simulink model "gridv1"  (R2021a)
settings: Solver=VariableStepAuto  StartTime=0.0  StopTime=inf  RelTol=1e-3
libraries: spsThreePhaseBreakerLib x12, spsMosfetLib x12, spsThreePhaseSeriesRLCLoadLib x10, spsMeanLib x6, pid_lib x5, simulink x4, spsPLL3phLib x4, spsThreePhaseVIMeasurementLib x4, spsAsynchronousMachineSIUnitsLib x2, spsDCVoltageSourceLib x2, spsFourierLib x2, spsGroundLib x2
(part 1 of 2)
settings Model: SimulationMode=accelerator  Creator=Ramadan B.M.S  LastModifiedBy=Ramadan B.M.S
settings SolverCC: ZeroCrossAlgorithm=Adaptive  AutoInsertRateTranBlk=on
settings DebuggingCC: IgnoredZcDiagnostic=none

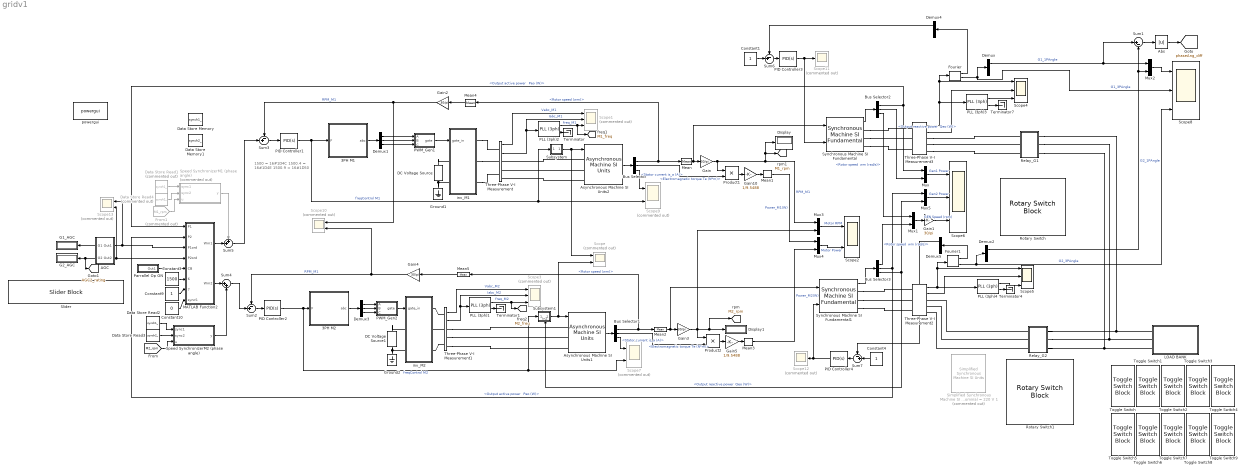
== system gridv1 ==
  note: 1500 = 16#1D4C
      | 1500.4 = 16#1D4E
      | 1500.9 = 16#1D50
  3PH M1 : Subsystem
  3PH M2 : Subsystem
  AGC : Subsystem
      settings: PortSchema="{\"entries\":[{\"content\":{\"sides\":[{\"content\":{\"connectorIds\":[\"Out3\",\"Out4\"]},\"type\":\"ConnectorPlacement.EquallySpacedRectSide\",\"uuid\":\"0458f88f-2a90-4e9d-a6e7-72d7481f8c74\"},{\"content\":{\"connectorIds\":[\"Out1\",\"Out2\"],\"side\":\"RIGHT\"},\"type\":\"ConnectorPlacement.EquallySpacedRectSide\",\"uuid\":\"40e75e7a-a838-46b0-adb7-8af141426c13\"},{\"content\":{\"connectorIds\":[],\"side\":\"TOP\"},\"type\":\"ConnectorPlacement.EquallySpacedRectSide\",\"uuid\":\"7ac7dab2-5483-477d-b4b4-330f83a557ce\"}]},\"type\":\"ConnectorPlacement.EquallySpacedConnector\",\"uuid\":\"5bf97401-9b0d-4cd2-ac22-a4057234a7d6\"}],\"packageUris\":[\"http://schema.mathworks.com/mf0/Connector/R2020b\"],\"version\":\"1.0\"}"
  Abs : Abs
  Asynchronous Machine SI Units1 : spsAsynchronousMachineSIUnitsLib/Asynchronous Machine SI Units  RotorType=Squirrel-cage  PresetModel="17:  20 HP (15KW)   400 V 50Hz 1460 RPM"  MechanicalLoad=Torque Tm  ShowDetailedParameters=on  ReferenceFrame=Rotor  Units=SI  MeasurementBus=off  NominalParameters=[1.5e+04 400 50]  VoltageRatio=1  Stator=[0.2147 0.000991]  Rotor=[0.2205 0.000991]  Cage1=[0.4155 0.002066]  Cage2=[0.4168 0.0003495]  Lm=0.06419  Mechanical=[0.102 0.009541 2]  PolePairs=2  InitialConditions=[0 0 0 0 0 0 0 0]  SimulateSaturation=off  Saturation=[14.03593122, 27.81365428, 53.79336849, 72.68890987, 97.98006896, 148.6815601, 215.7428561, 302.9841135, 428.7778367 ; 230, 322, 414, 460, 506, 552, 598, 644, 690]  LoadFlowParameters=1492000  TsPowergui=0  TsBlock=-1  IterativeModel=Trapezoidal non iterative  IterativeDiscreteModel=Trapezoidal robust  Pmec=0  mask(Asynchronous Machine){}
      mask Display: image('M2.jpg'); % Use "Edit Image" on toolstrip to change.
  Asynchronous Machine SI Units2 : spsAsynchronousMachineSIUnitsLib/Asynchronous Machine SI Units  RotorType=Squirrel-cage  PresetModel="17:  20 HP (15KW)   400 V 50Hz 1460 RPM"  MechanicalLoad=Torque Tm  ShowDetailedParameters=on  ReferenceFrame=Rotor  Units=SI  MeasurementBus=off  NominalParameters=[1.5e+04 400 50]  VoltageRatio=1  Stator=[0.2147 0.000991]  Rotor=[0.2205 0.000991]  Cage1=[0.4155 0.002066]  Cage2=[0.4168 0.0003495]  Lm=0.06419  Mechanical=[0.102 0.009541 2]  PolePairs=2  InitialConditions=[0 0 0 0 0 0 0 0]  SimulateSaturation=off  Saturation=[14.03593122, 27.81365428, 53.79336849, 72.68890987, 97.98006896, 148.6815601, 215.7428561, 302.9841135, 428.7778367 ; 230, 322, 414, 460, 506, 552, 598, 644, 690]  LoadFlowParameters=1492000  TsPowergui=0  TsBlock=-1  IterativeModel=Trapezoidal non iterative  IterativeDiscreteModel=Trapezoidal robust  Pmec=0  mask(Asynchronous Machine){}
      mask Display: image('M1.jpg'); % Use "Edit Image" on toolstrip to change.
  Bus Selector : BusSelector  OutputSignals=Mechanical.Rotor speed (wm),Mechanical.Electromagnetic torque Te (N*m),Stator measurements.Stator current is_a (A)
  Bus Selector1 : BusSelector  OutputSignals=Mechanical.Rotor speed (wm),Mechanical.Electromagnetic torque Te (N*m),Stator measurements.Stator current is_a (A)
  Bus Selector2 : BusSelector  OutputSignals="Output active power   Peo (W),Output reactive power  Qeo (W),Mechanical.Rotor speed  wm (rad/s)"
  Bus Selector3 : BusSelector  OutputSignals="Mechanical.Rotor speed  wm (rad/s),Output active power   Peo (W),Output reactive power  Qeo (W)"
  Constant1 : Constant
  Constant10 : Constant  Value=0
  Constant3 : Constant  Value=1500
  Constant4 : Constant
  Constant9 : Constant
  DC Voltage Source : spsDCVoltageSourceLib/DC Voltage Source  Amplitude=566  Measurements=None
  DC Voltage Source1 : spsDCVoltageSourceLib/DC Voltage Source  Amplitude=566  Measurements=None
  Data Store Memory : DataStoreMemory  DataStoreName=synch1_  ReadBeforeWriteMsg=warning  WriteAfterWriteMsg=warning  WriteAfterReadMsg=warning  ShowAdditionalParam=off
  Data Store Memory1 : DataStoreMemory  DataStoreName=synch2_  ReadBeforeWriteMsg=warning  WriteAfterWriteMsg=warning  WriteAfterReadMsg=warning  ShowAdditionalParam=off
  Data Store Read1 : DataStoreRead  Commented=on  DataStoreName=synch1_  IndexOptions=Index vector (dialog)  Indices=1  OutputSizes=1
  Data Store Read2 : DataStoreRead  DataStoreName=synch1_  IndexOptions=Index vector (dialog)  Indices=1  OutputSizes=1
  Data Store Read3 : DataStoreRead  DataStoreName=synch2_  IndexOptions=Index vector (dialog)  Indices=1  OutputSizes=1
  Data Store Read4 : DataStoreRead  Commented=on  DataStoreName=synch2_  IndexOptions=Index vector (dialog)  Indices=1  OutputSizes=1
  Demux{,1..5} (6 alike) : Demux  Outputs=3
  Display : Display
  Display1 : Display
  Fourier : spsFourierLib/Fourier  Freq=50  n=1  InInit=[0, 0]  Ts=0
      settings: SourceProductBaseCode=PS
  Fourier1 : spsFourierLib/Fourier  Freq=50  n=1  InInit=[0, 0]  Ts=0
      settings: SourceProductBaseCode=PS
  From1 : From  Commented=on  GotoTag=M1_rpm  TagVisibility=global
  G1_AGC : Display
      settings: Decimation=100
  G2_AGC : Display
      settings: Decimation=100
  Gain{,1..4} (5 alike) : Gain  Gain=30/pi
  Gain10 : Gain  Gain=1/9.5488
  Gain5 : Gain  Gain=1/9.5488
  Ground1 : spsGroundLib/Ground  LConnTagsString=a
  Ground2 : spsGroundLib/Ground  LConnTagsString=a
  LOAD BANK : Subsystem
  MATLAB Function2 : MATLAB Function  TreatAsAtomicUnit=on
  Mean{,1..3} (4 alike) : spsMeanLib/Mean  Freq=1  Vinit=0  Ts=0
  Mean4 : spsMeanLib/Mean  Freq=10  Vinit=0  Ts=0
  Mean5 : spsMeanLib/Mean  Freq=10  Vinit=0  Ts=0
  Mux{,1..5} (6 alike) : Mux  Inputs=2
  PID Controller1 : pid_lib/PID Controller  Controller=PID  Form=Parallel  TimeDomain=Continuous-time  UseExternalTs=off  SampleTime=-1  IntegratorMethod=Forward Euler  FilterMethod=Forward Euler  ControllerParametersSource=internal  P=0.06  I=0.12  D=0  UseFilter=on  N=100  TunerSelectOption=Transfer Function Based (PID Tuner App)  ZeroCross=off  InitialConditionSource=internal  InitialConditionForIntegrator=0  InitialConditionForFilter=0  DifferentiatorICPrevScaledInput=0  ExternalReset=none  TrackingMode=off  Kt=1  LimitOutput=on  SatLimitsSource=internal  UpperSaturationLimit=52.5  LowerSaturationLimit=0  LinearizeAsGain=on  AntiWindupMode=back-calculation  Kb=1  POutMin=[]  POutMax=[]  IOutMin=[]  IOutMax=[]  DOutMin=[]  DOutMax=[]  NOutMin=[]  NOutMax=[]  SumOutMin=[]  SumOutMax=[]  SaturationOutMin=[]  SaturationOutMax=[]  PParamMin=[]  PParamMax=[]  IParamMin=[]  IParamMax=[]  DParamMin=[]  DParamMax=[]  NParamMin=[]  NParamMax=[]  KbParamMin=[]  KbParamMax=[]  KtParamMin=[]  KtParamMax=[]  KbOutMin=[]  KbOutMax=[]  KtOutMin=[]  KtOutMax=[]  IntegratorOutMin=[]  IntegratorOutMax=[]  FilterOutMin=[]  FilterOutMax=[]  SumI1OutMin=[]  SumI1OutMax=[]  SumI2OutMin=[]  SumI2OutMax=[]  SumI3OutMin=[]  SumI3OutMax=[]  SumI4OutMin=[]  SumI4OutMax=[]  SumDOutMin=[]  SumDOutMax=[]  DifferentiatorOutMin=[]  DifferentiatorOutMax=[]  FilterDiffOutCoefMin=[]  FilterDiffOutCoefMax=[]  ReciprocalOutMin=[]  ReciprocalOutMax=[]  SumDenOutMin=[]  SumDenOutMax=[]  SumNumOutMin=[]  SumNumOutMax=[]  DivideOutMin=[]  DivideOutMax=[]  UdiffTsProdOutMin=[]  UdiffTsProdOutMax=[]  NTsProdOutMin=[]  NTsProdOutMax=[]  UintegralTsProdOutMin=[]  UintegralTsProdOutMax=[]  UngainTsProdOutMin=[]  UngainTsProdOutMax=[]  IntegratorContinuousStateAttributes=''  IntegratorStateMustResolveToSignalObject=off  IntegratorRTWStateStorageClass=Auto  FilterContinuousStateAttributes=''  FilterStateMustResolveToSignalObject=off  FilterRTWStateStorageClass=Auto  ParallelPVariant=InternalParameters  IdealPVariant=Disabled  IVariant=InternalParameters  DVariant=InternalParameters  IntegratorVariant=Continuous  SatVariant=Enabled  AWVariant=BackCalculation  PCopyVariant=Disabled  TRVariant=Disabled  FdbkBlocksVariant=Forward  IdealPFdbkVariant=Disabled  SatFdbkVariant=Disabled  DerivativeFilterVariant=ContFilter  NVariant=InternalParameters  NCopyVariant=Disabled  FilterICVariant=InternalICsFilter  IntegratorICVariant=InternalICs  ExternalResetVariant=Disabled  TRSumVariant=Passthrough  SumFdbkVariant=Disabled  SumVariant=Sum_PID  TsampFilterVariant=InternalTs  TsampNgainVariant=Passthrough  TsampIntegralVariant=Passthrough  ExternalSaturationOutDataTypeStr=Inherit: Same as second input
  PID Controller2 : pid_lib/PID Controller  Controller=PID  Form=Parallel  TimeDomain=Continuous-time  UseExternalTs=off  SampleTime=-1  IntegratorMethod=Forward Euler  FilterMethod=Forward Euler  ControllerParametersSource=internal  P=0.06  I=0.12  D=0  UseFilter=on  N=100  TunerSelectOption=Transfer Function Based (PID Tuner App)  ZeroCross=off  InitialConditionSource=internal  InitialConditionForIntegrator=0  InitialConditionForFilter=0  DifferentiatorICPrevScaledInput=0  ExternalReset=none  TrackingMode=off  Kt=1  LimitOutput=on  SatLimitsSource=internal  UpperSaturationLimit=52.5  LowerSaturationLimit=0  LinearizeAsGain=on  AntiWindupMode=back-calculation  Kb=1  POutMin=[]  POutMax=[]  IOutMin=[]  IOutMax=[]  DOutMin=[]  DOutMax=[]  NOutMin=[]  NOutMax=[]  SumOutMin=[]  SumOutMax=[]  SaturationOutMin=[]  SaturationOutMax=[]  PParamMin=[]  PParamMax=[]  IParamMin=[]  IParamMax=[]  DParamMin=[]  DParamMax=[]  NParamMin=[]  NParamMax=[]  KbParamMin=[]  KbParamMax=[]  KtParamMin=[]  KtParamMax=[]  KbOutMin=[]  KbOutMax=[]  KtOutMin=[]  KtOutMax=[]  IntegratorOutMin=[]  IntegratorOutMax=[]  FilterOutMin=[]  FilterOutMax=[]  SumI1OutMin=[]  SumI1OutMax=[]  SumI2OutMin=[]  SumI2OutMax=[]  SumI3OutMin=[]  SumI3OutMax=[]  SumI4OutMin=[]  SumI4OutMax=[]  SumDOutMin=[]  SumDOutMax=[]  DifferentiatorOutMin=[]  DifferentiatorOutMax=[]  FilterDiffOutCoefMin=[]  FilterDiffOutCoefMax=[]  ReciprocalOutMin=[]  ReciprocalOutMax=[]  SumDenOutMin=[]  SumDenOutMax=[]  SumNumOutMin=[]  SumNumOutMax=[]  DivideOutMin=[]  DivideOutMax=[]  UdiffTsProdOutMin=[]  UdiffTsProdOutMax=[]  NTsProdOutMin=[]  NTsProdOutMax=[]  UintegralTsProdOutMin=[]  UintegralTsProdOutMax=[]  UngainTsProdOutMin=[]  UngainTsProdOutMax=[]  IntegratorContinuousStateAttributes=''  IntegratorStateMustResolveToSignalObject=off  IntegratorRTWStateStorageClass=Auto  FilterContinuousStateAttributes=''  FilterStateMustResolveToSignalObject=off  FilterRTWStateStorageClass=Auto  ParallelPVariant=InternalParameters  IdealPVariant=Disabled  IVariant=InternalParameters  DVariant=InternalParameters  IntegratorVariant=Continuous  SatVariant=Enabled  AWVariant=BackCalculation  PCopyVariant=Disabled  TRVariant=Disabled  FdbkBlocksVariant=Forward  IdealPFdbkVariant=Disabled  SatFdbkVariant=Disabled  DerivativeFilterVariant=ContFilter  NVariant=InternalParameters  NCopyVariant=Disabled  FilterICVariant=InternalICsFilter  IntegratorICVariant=InternalICs  ExternalResetVariant=Disabled  TRSumVariant=Passthrough  SumFdbkVariant=Disabled  SumVariant=Sum_PID  TsampFilterVariant=InternalTs  TsampNgainVariant=Passthrough  TsampIntegralVariant=Passthrough  ExternalSaturationOutDataTypeStr=Inherit: Same as second input
  PID Controller3 : pid_lib/PID Controller  Controller=PID  Form=Parallel  TimeDomain=Continuous-time  UseExternalTs=off  SampleTime=-1  IntegratorMethod=Forward Euler  FilterMethod=Forward Euler  ControllerParametersSource=internal  P=10  I=17  D=0  UseFilter=on  N=100  TunerSelectOption=Transfer Function Based (PID Tuner App)  ZeroCross=off  InitialConditionSource=internal  InitialConditionForIntegrator=0  InitialConditionForFilter=0  DifferentiatorICPrevScaledInput=0  ExternalReset=none  TrackingMode=off  Kt=1  LimitOutput=on  SatLimitsSource=internal  UpperSaturationLimit=15  LowerSaturationLimit=0  LinearizeAsGain=on  AntiWindupMode=back-calculation  Kb=1  POutMin=[]  POutMax=[]  IOutMin=[]  IOutMax=[]  DOutMin=[]  DOutMax=[]  NOutMin=[]  NOutMax=[]  SumOutMin=[]  SumOutMax=[]  SaturationOutMin=[]  SaturationOutMax=[]  PParamMin=[]  PParamMax=[]  IParamMin=[]  IParamMax=[]  DParamMin=[]  DParamMax=[]  NParamMin=[]  NParamMax=[]  KbParamMin=[]  KbParamMax=[]  KtParamMin=[]  KtParamMax=[]  KbOutMin=[]  KbOutMax=[]  KtOutMin=[]  KtOutMax=[]  IntegratorOutMin=[]  IntegratorOutMax=[]  FilterOutMin=[]  FilterOutMax=[]  SumI1OutMin=[]  SumI1OutMax=[]  SumI2OutMin=[]  SumI2OutMax=[]  SumI3OutMin=[]  SumI3OutMax=[]  SumI4OutMin=[]  SumI4OutMax=[]  SumDOutMin=[]  SumDOutMax=[]  DifferentiatorOutMin=[]  DifferentiatorOutMax=[]  FilterDiffOutCoefMin=[]  FilterDiffOutCoefMax=[]  ReciprocalOutMin=[]  ReciprocalOutMax=[]  SumDenOutMin=[]  SumDenOutMax=[]  SumNumOutMin=[]  SumNumOutMax=[]  DivideOutMin=[]  DivideOutMax=[]  UdiffTsProdOutMin=[]  UdiffTsProdOutMax=[]  NTsProdOutMin=[]  NTsProdOutMax=[]  UintegralTsProdOutMin=[]  UintegralTsProdOutMax=[]  UngainTsProdOutMin=[]  UngainTsProdOutMax=[]  IntegratorContinuousStateAttributes=''  IntegratorStateMustResolveToSignalObject=off  IntegratorRTWStateStorageClass=Auto  FilterContinuousStateAttributes=''  FilterStateMustResolveToSignalObject=off  FilterRTWStateStorageClass=Auto  ParallelPVariant=InternalParameters  IdealPVariant=Disabled  IVariant=InternalParameters  DVariant=InternalParameters  IntegratorVariant=Continuous  SatVariant=Enabled  AWVariant=BackCalculation  PCopyVariant=Disabled  TRVariant=Disabled  FdbkBlocksVariant=Forward  IdealPFdbkVariant=Disabled  SatFdbkVariant=Disabled  DerivativeFilterVariant=ContFilter  NVariant=InternalParameters  NCopyVariant=Disabled  FilterICVariant=InternalICsFilter  IntegratorICVariant=InternalICs  ExternalResetVariant=Disabled  TRSumVariant=Passthrough  SumFdbkVariant=Disabled  SumVariant=Sum_PID  TsampFilterVariant=InternalTs  TsampNgainVariant=Passthrough  TsampIntegralVariant=Passthrough  ExternalSaturationOutDataTypeStr=Inherit: Same as second input
  PID Controller4 : pid_lib/PID Controller  Controller=PID  Form=Parallel  TimeDomain=Continuous-time  UseExternalTs=off  SampleTime=-1  IntegratorMethod=Forward Euler  FilterMethod=Forward Euler  ControllerParametersSource=internal  P=10  I=17  D=0  UseFilter=on  N=100  TunerSelectOption=Transfer Function Based (PID Tuner App)  ZeroCross=off  InitialConditionSource=internal  InitialConditionForIntegrator=0  InitialConditionForFilter=0  DifferentiatorICPrevScaledInput=0  ExternalReset=none  TrackingMode=off  Kt=1  LimitOutput=on  SatLimitsSource=internal  UpperSaturationLimit=15  LowerSaturationLimit=0  LinearizeAsGain=on  AntiWindupMode=back-calculation  Kb=1  POutMin=[]  POutMax=[]  IOutMin=[]  IOutMax=[]  DOutMin=[]  DOutMax=[]  NOutMin=[]  NOutMax=[]  SumOutMin=[]  SumOutMax=[]  SaturationOutMin=[]  SaturationOutMax=[]  PParamMin=[]  PParamMax=[]  IParamMin=[]  IParamMax=[]  DParamMin=[]  DParamMax=[]  NParamMin=[]  NParamMax=[]  KbParamMin=[]  KbParamMax=[]  KtParamMin=[]  KtParamMax=[]  KbOutMin=[]  KbOutMax=[]  KtOutMin=[]  KtOutMax=[]  IntegratorOutMin=[]  IntegratorOutMax=[]  FilterOutMin=[]  FilterOutMax=[]  SumI1OutMin=[]  SumI1OutMax=[]  SumI2OutMin=[]  SumI2OutMax=[]  SumI3OutMin=[]  SumI3OutMax=[]  SumI4OutMin=[]  SumI4OutMax=[]  SumDOutMin=[]  SumDOutMax=[]  DifferentiatorOutMin=[]  DifferentiatorOutMax=[]  FilterDiffOutCoefMin=[]  FilterDiffOutCoefMax=[]  ReciprocalOutMin=[]  ReciprocalOutMax=[]  SumDenOutMin=[]  SumDenOutMax=[]  SumNumOutMin=[]  SumNumOutMax=[]  DivideOutMin=[]  DivideOutMax=[]  UdiffTsProdOutMin=[]  UdiffTsProdOutMax=[]  NTsProdOutMin=[]  NTsProdOutMax=[]  UintegralTsProdOutMin=[]  UintegralTsProdOutMax=[]  UngainTsProdOutMin=[]  UngainTsProdOutMax=[]  IntegratorContinuousStateAttributes=''  IntegratorStateMustResolveToSignalObject=off  IntegratorRTWStateStorageClass=Auto  FilterContinuousStateAttributes=''  FilterStateMustResolveToSignalObject=off  FilterRTWStateStorageClass=Auto  ParallelPVariant=InternalParameters  IdealPVariant=Disabled  IVariant=InternalParameters  DVariant=InternalParameters  IntegratorVariant=Continuous  SatVariant=Enabled  AWVariant=BackCalculation  PCopyVariant=Disabled  TRVariant=Disabled  FdbkBlocksVariant=Forward  IdealPFdbkVariant=Disabled  SatFdbkVariant=Disabled  DerivativeFilterVariant=ContFilter  NVariant=InternalParameters  NCopyVariant=Disabled  FilterICVariant=InternalICsFilter  IntegratorICVariant=InternalICs  ExternalResetVariant=Disabled  TRSumVariant=Passthrough  SumFdbkVariant=Disabled  SumVariant=Sum_PID  TsampFilterVariant=InternalTs  TsampNgainVariant=Passthrough  TsampIntegralVariant=Passthrough  ExternalSaturationOutDataTypeStr=Inherit: Same as second input
  PLL (3ph){1..4} (4 alike) : spsPLL3phLib/PLL (3ph)  Fmin=45  Par_Init=[0, 1]  ParK=[180, 3800, 1]  TcD=1e-4  MaxRateChangeFreq=12  FilterCutOffFreq=25  Ts=0  AGC=on
  PWM_Gen1 : Subsystem
  PWM_Gen2 : Subsystem
  Parrallel Op ON : Subsystem
  Product1 : Product
  Product2 : Product
  Relay_G1 : Subsystem
  Relay_G2 : Subsystem
  Rotary Switch : RotarySwitchBlock
      settings: Values={{'OPEN', 'CLOSE'}, [0 1]}
  Rotary Switch1 : RotarySwitchBlock
      settings: Values={{'OPEN', 'CLOSE'}, [0 1]}
  Scope{,7,9..10,13} (5 alike) : Scope  Commented=on  NumInputPorts=2
  Scope1 : Scope  Commented=on  NumInputPorts=3
  Scope11 : Scope  Commented=on
  Scope12 : Scope  Commented=on
  Scope2 : Scope  NumInputPorts=2
  Scope3 : Scope  Commented=on  NumInputPorts=3
  Scope{4..6,8} (4 alike) : Scope  NumInputPorts=3
  Simplified Synchronous Machine SI Units If nominal  = 1.8 A Xs = 18.85 Ohm a 1800 rpm Ls = 0.05 H Laf = 0.4584 H Ea_LL nominal = 220 V 1 : spsSimplifiedSynchronousMachineSIUnitsLib/Simplified Synchronous Machine SI Units  Commented=on  ConnectionType=3-wire Y  MechanicalLoad=Speed w  MeasurementBus=off  NominalParameters=[15000 400 50]  Mechanical=[1e6 0 2]  InternalRL=[0.01 0.01]  InitialConditions="[ 0,0   0,0,0   0,0,0 ]"  IterativeDiscreteModel=Trapezoidal robust  TsBlock=-1  TsPowergui=0  LoadFlowParameters=[1,0,0,0,0]  Units=1  BusType=PV  Pref=0  Qref=0  Qmin=-inf  Qmax=+inf  PLF=0  QLF=0  mask(Simplified Synchronous Machine){}
      settings: SourceProductBaseCode=PS
      mask Display: image('G2.jpg'); % Use "Edit Image" on toolstrip to change.
  Slider : SliderBlock  TickInterval=10
  Speed SynchronizerM1 (phase angle) : MATLAB Function  Commented=on  TreatAsAtomicUnit=on
  Speed SynchronizerM2 (phase angle) : MATLAB Function  TreatAsAtomicUnit=on
  Subsystem : Subsystem
  Subsystem1 : Subsystem
      settings: PortSchema="{\"entries\":[{\"content\":{\"sides\":[{\"content\":{\"connectorIds\":[\"In1\"]},\"type\":\"ConnectorPlacement.EquallySpacedRectSide\",\"uuid\":\"6fb75f93-f453-4c8c-8eb2-b078f2ee4494\"},{\"content\":{\"connectorIds\":[\"Out1\"],\"side\":\"RIGHT\"},\"type\":\"ConnectorPlacement.EquallySpacedRectSide\",\"uuid\":\"6ec336d8-76a4-4c07-bc41-67ee684e5bd8\"},{\"content\":{\"connectorIds\":[],\"side\":\"TOP\"},\"type\":\"ConnectorPlacement.EquallySpacedRectSide\",\"uuid\":\"24ce01c0-9e7f-4b6f-9b18-6c8c2670b010\"},{\"content\":{\"connectorIds\":[\"In2\"],\"side\":\"BOTTOM\"},\"type\":\"ConnectorPlacement.EquallySpacedRectSide\",\"uuid\":\"901aa75b-c78e-4bda-b9b4-99ea4194a71a\"}]},\"type\":\"ConnectorPlacement.EquallySpacedConnector\",\"uuid\":\"a6afde9e-346d-4066-a3a3-61c85561d5e0\"}],\"packageUris\":[\"http://schema.mathworks.com/mf0/Connector/R2020b\"],\"version\":\"1.0\"}"
  Sum1 : Sum  Inputs=|+-
  Sum{2..3,6..7} (4 alike) : Sum  Inputs=-+|
  Sum4 : Sum  Inputs=|++
  Sum5 : Sum  Inputs=++|
  Synchronous Machine SI Fundamental : spsSynchronousMachineSIFundamentalLib/Synchronous Machine SI Fundamental  PresetModel=02: 50Hz 400V 16kVA 1500RPM  MechanicalLoad=Speed w  ShowDetailedParameters=on  RotorType=Salient-pole  Units=SI fundamental parameters  MeasurementBus=off  NominalParameters=[1.6e+04 400 50]  Stator=[0.645 0.002228 0.05297 0.02518]  Field=[0.3968 0.005492]  Dampers2=[ 0.0664, 1.387e-3, 0.0292, 6.896e-4, 7.907e-3, 2.477e-3]  Dampers1=[0.9843 0.003371 1.545 0.004906]  Mechanical=[0.1278 0.013 2]  PolePairs=2  InitialConditions="[ 0  0  0  0  0  0  0  0  70.3192 ]"  SetSaturation=off  Saturation=[695.64,774.7,917.5,1001.6,1082.2,1175.9,1293.6,1430.2,1583.7;9660,10623,12243,13063,13757,14437,15180,15890,16567]  DisplayVfd=off  LoadFlowParameters=[1,0,0,0,0]  TsPowergui=0  TsBlock=-1  IterativeModel=Trapezoidal non iterative  IterativeDiscreteModel=Trapezoidal robust  BusType=PV  Pref=0  Qref=0  Qmin=-inf  Qmax=inf  PLF=0  QLF=0
      settings: SourceProductBaseCode=PS
  Synchronous Machine SI Fundamental1 : spsSynchronousMachineSIFundamentalLib/Synchronous Machine SI Fundamental  PresetModel=02: 50Hz 400V 16kVA 1500RPM  MechanicalLoad=Speed w  ShowDetailedParameters=on  RotorType=Salient-pole  Units=SI fundamental parameters  MeasurementBus=off  NominalParameters=[1.6e+04 400 50]  Stator=[0.645 0.002228 0.05297 0.02518]  Field=[0.3968 0.005492]  Dampers2=[ 0.0664, 1.387e-3, 0.0292, 6.896e-4, 7.907e-3, 2.477e-3]  Dampers1=[0.9843 0.003371 1.545 0.004906]  Mechanical=[0.1278 0.013 2]  PolePairs=2  InitialConditions="[ 0  0  0  0  0  0  0  0  70.3192 ]"  SetSaturation=off  Saturation=[695.64,774.7,917.5,1001.6,1082.2,1175.9,1293.6,1430.2,1583.7;9660,10623,12243,13063,13757,14437,15180,15890,16567]  DisplayVfd=off  LoadFlowParameters=[1,0,0,0,0]  TsPowergui=0  TsBlock=-1  IterativeModel=Trapezoidal non iterative  IterativeDiscreteModel=Trapezoidal robust  BusType=PV  Pref=0  Qref=0  Qmin=-inf  Qmax=inf  PLF=0  QLF=0
      settings: SourceProductBaseCode=PS
  Terminator{,1,4,7} (4 alike) : Terminator
  Three-Phase V-I Measurement{,1..3} (4 alike) : spsThreePhaseVIMeasurementLib/Three-Phase V-I Measurement  VoltageMeasurement=phase-to-phase  SetLabelV=off  LabelV=Vabc  Vpu=off  VpuLL=on  CurrentMeasurement=yes  SetLabelI=off  LabelI=Iabc  Ipu=off  Pbase=100e6  Vbase=400  OutputType=Complex  PhasorSimulation=off  PSBequivalent=0
  Toggle Switch{,1..9} (10 alike) : ToggleSwitchBlock
      settings: Values={{'Off', 'On'}, [0 1]}
  inv_M1 : Subsystem
  inv_M2 : Subsystem
  powergui : spspowerguiLib/powergui  Priority=1  SimulationMode=Discrete  SampleTime=5e-5  frequency=60  Iterations=50  frequencyindice=0  Pbase=100e6  ErrMax=1e-4  UnitsV=kV  UnitsW=MW  buscounter=0  FunctionMessages=off  echomessages=off  EnableUseOfTLC=off  CurrentSourceSwitches=off  DisableSnubberDevices=off  DisableRonSwitches=off  DisableVfSwitches=off  DisplayEquations=off  AutomaticDiscreteSolvers=off  SolverType=Tustin/Backward Euler (TBE)  Interpol=off  ExternalGateDelay=off  methode=off  Ts=100  x0status=blocks  SPID=on  SwTol=0  HookPort=off  NonlinearTolerance=1e-4  nMaxIteration=100  ContinueOnMaxIteration=off  RestoreLinks=warning  ResistiveCurrentMeasurement=off  Frange=[0:2:500]  Ylog=off  Xlog=on  ShowGrid=off  save=off  variable=ZData  structure=0  ZoomFFT=off  StartTime=0.0  cycles=1  DisplayStyle=1  fundamental=60  FreqAxis=off  MaxFrequency=1000  frequencyindicesteady=1  RmsSteady=1  display=off
  tag scope: AGC2_rating=global, M1_freq=global, M1_rpm=global, M2_freq=global, M2_rpm=global, phaseAng_diff=global
  wires:
  Asynchronous Machine SI Units2/1 -> Bus Selector/1
  3PH M1/1(abc) -> Demux1/1
  Demux1/2 -> PWM_Gen1/2(B)
  Demux1/1 -> PWM_Gen1/1(A)
  Subsystem/1(Out1) -> Scope/1, Asynchronous Machine SI Units2/1
  Three-Phase V-I Measurement/1 -> Scope1/1  "Vabc_M1"
  Three-Phase V-I Measurement/2 -> PLL (3ph)2/1, Scope1/2  "Iabc_M1"
  Product1/1 -> Gain10/1
  Gain10/1 -> Mean1/1
  Bus Selector/2 -> Product1/2  "<Electromagnetic torque Te (N*m)>"
  Bus Selector/3 -> Scope9/1  "<Stator current is_a (A)>"
  Mean1/1 -> Mux4/1  "Power_M1(W)"
  Mean3/1 -> Mux4/2  "Power_M2(W)"
  Demux3/2 -> PWM_Gen2/2(B)
  Product2/1 -> Gain5/1
  Gain5/1 -> Mean3/1
  Subsystem1/1(Out1) -> Scope/2, Asynchronous Machine SI Units1/1
  3PH M2/1(abc) -> Demux3/1
  Demux3/3 -> PWM_Gen2/3(C)
  Bus Selector1/2 -> Product2/2  "<Electromagnetic torque Te (N*m)>"
  Asynchronous Machine SI Units1/1 -> Bus Selector1/1
  Bus Selector1/3 -> Scope7/1  "<Stator current is_a (A)>"
  Demux3/1 -> PWM_Gen2/1(A)
  PLL (3ph)2/1 -> [M1_freq], Scope1/3  "freq_M1"
  Synchronous Machine SI Fundamental/1 -> Bus Selector2/1
  PLL (3ph)3/1 -> Scope4/3
  Sum2/1 -> PID Controller2/1
  PID Controller2/1 -> Scope7/2, Subsystem1/1(In1), 3PH M2/1(F)  "freqControl M2"
  Synchronous Machine SI Fundamental1/1 -> Bus Selector3/1
  Three-Phase V-I Measurement2/2 -> Scope5/2
  PLL (3ph)4/1 -> Scope5/3
  Three-Phase V-I Measurement2/1 -> Fourier1/1, Scope5/1, PLL (3ph)4/1
  Fourier/2 -> Scope8/2, Demux/1  "G1_3PAngle"
  Fourier1/2 -> Scope8/3, Demux2/1  "G2_3PAngle"
  PID Controller1/1 -> 3PH M1/1(F), Subsystem/1(In1), Scope9/2  "freqControl M1"
  Bus Selector/1 -> Mean/1, Mean4/1  "<Rotor speed (wm)>"
  Bus Selector1/1 -> Mean5/1, Mean2/1  "<Rotor speed (wm)>"
  Sum3/1 -> PID Controller1/1
  Three-Phase V-I Measurement1/1 -> Scope3/1  "Vabc_M2"
  PLL (3ph)1/1 -> [M2_freq], Scope3/3  "freq_M2"
  Gain/1 -> Mux3/1, Display/1, [M1_rpm], Product1/1  "RPM_M1"
  Three-Phase V-I Measurement1/2 -> PLL (3ph)1/1, Scope3/2  "Iabc_M2"
  PLL (3ph)2/2 -> Terminator/1
  PLL (3ph)1/2 -> Terminator1/1
  Mean2/1 -> Synchronous Machine SI Fundamental1/1, Gain3/1
  Mean/1 -> Synchronous Machine SI Fundamental/1, Gain/1
  Gain1/1 -> Scope6/3  "GEN Speed (rpm)"
  Mux/1 -> Scope6/1  "Gen1 Power"
  Mux1/1 -> Gain1/1
  Bus Selector2/1 -> MATLAB Function2/1(P1), Mux/1  "<Output active power   Peo (W)>"
  Demux/1 -> Mux2/1, Sum1/1  "G1_1PAngle"
  Mux2/1 -> Scope8/1
  Demux2/1 -> Sum1/2, Mux2/2  "G2_1PAngle"
  PWM_Gen2/1(gate) -> inv_M2/1(gate_in)
  PWM_Gen1/1(gate) -> inv_M1/1(gate_in)
  Demux1/3 -> PWM_Gen1/3(C)
  Mux3/1 -> Scope2/1  "Motor RPM"
  Mux4/1 -> Scope2/2  "Motor Power"
  PID Controller3/1 -> Synchronous Machine SI Fundamental/2, Scope11/1
  PID Controller4/1 -> Synchronous Machine SI Fundamental1/2, Scope12/1
  Constant3/1 -> MATLAB Function2/6(userG1)
  Constant9/1 -> MATLAB Function2/7(userG2)
  Constant10/1 -> MATLAB Function2/8(syncS)
  Sum1/1 -> Abs/1
  Abs/1 -> [phaseAng_diff]
  Sum4/1 -> Sum2/2
  Speed SynchronizerM2 (phase angle)/1(y) -> Sum4/2
  Gain3/1 -> Mux3/2, [M2_rpm], Display1/1, Product2/1
  [M2_rpm] -> Speed SynchronizerM2 (phase angle)/3(u)
  MATLAB Function2/1(Wm1) -> Sum5/2
  Sum5/1 -> Sum3/2
  Speed SynchronizerM1 (phase angle)/1(y) -> Sum5/1
  Parrallel Op ON/1(Out1) -> MATLAB Function2/5(CB)
  Data Store Read2/1 -> Speed SynchronizerM2 (phase angle)/1(sync1)
  Data Store Read3/1 -> Speed SynchronizerM2 (phase angle)/2(sync2)
  Data Store Read1/1 -> Speed SynchronizerM1 (phase angle)/1(sync1)
  Data Store Read4/1 -> Speed SynchronizerM1 (phase angle)/2(sync2)
  From1/1 -> Speed SynchronizerM1 (phase angle)/3(u)
  PLL (3ph)4/2 -> Terminator4/1
  PLL (3ph)3/2 -> Terminator7/1
  AGC/1(Out1) -> MATLAB Function2/3(P1ord), Scope13/1
  AGC/2(Out2) -> MATLAB Function2/4(P2ord), Scope13/2
  AGC/3(G1) -> G1_AGC/1
  AGC/4(G2) -> [AGC2_rating], G2_AGC/1
  Gain2/1 -> Scope10/1, Sum3/1  "RPM_M1"
  Gain4/1 -> Scope10/2, Sum2/1  "RPM_M1"
  Mean4/1 -> Gain2/1
  Mean5/1 -> Gain4/1
  Three-Phase V-I Measurement3/1 -> PLL (3ph)3/1, Scope4/1, Fourier/1
  Three-Phase V-I Measurement3/2 -> Scope4/2
  Fourier/1 -> Demux4/1
  Constant1/1 -> Sum6/2
  Sum6/1 -> PID Controller3/1
  Demux4/1 -> Sum6/1
  Constant4/1 -> Sum7/2
  Demux5/1 -> Sum7/1
  Sum7/1 -> PID Controller4/1
  Fourier1/1 -> Demux5/1
  Bus Selector2/3 -> Mux1/1  "<Rotor speed  wm (rad/s)>"
  Bus Selector3/1 -> Mux1/2  "<Rotor speed  wm (rad/s)>"
  Bus Selector2/2 -> Mux/2  "<Output reactive power  Qeo (W)>"
  Mux5/1 -> Scope6/2  "Gen2 Power"
  Bus Selector3/2 -> Mux5/1, MATLAB Function2/2(P2)  "<Output active power   Peo (W)>"
  Bus Selector3/3 -> Mux5/2, Subsystem1/2(In2)  "<Output reactive power  Qeo (W)>"
  MATLAB Function2/2(Wm2) -> Sum4/1
  connections:
  Asynchronous Machine SI Units2/LConn1 -- Three-Phase V-I Measurement/RConn1
  Asynchronous Machine SI Units2/LConn2 -- Three-Phase V-I Measurement/RConn2
  Asynchronous Machine SI Units2/LConn3 -- Three-Phase V-I Measurement/RConn3
  Synchronous Machine SI Fundamental/RConn1 -- Three-Phase V-I Measurement3/LConn1
  Synchronous Machine SI Fundamental/RConn3 -- Three-Phase V-I Measurement3/LConn3
  Synchronous Machine SI Fundamental/RConn2 -- Three-Phase V-I Measurement3/LConn2
  Synchronous Machine SI Fundamental1/RConn3 -- Three-Phase V-I Measurement2/LConn3
  Synchronous Machine SI Fundamental1/RConn1 -- Three-Phase V-I Measurement2/LConn1
  Synchronous Machine SI Fundamental1/RConn2 -- Three-Phase V-I Measurement2/LConn2
  Three-Phase V-I Measurement1/RConn1 -- Asynchronous Machine SI Units1/LConn1
  Three-Phase V-I Measurement1/RConn2 -- Asynchronous Machine SI Units1/LConn2
  Three-Phase V-I Measurement1/RConn3 -- Asynchronous Machine SI Units1/LConn3
  Ground2/LConn1 -- DC Voltage Source1/LConn1 -- inv_M2/LConn2
  Three-Phase V-I Measurement1/LConn1 -- inv_M2/RConn1
  DC Voltage Source1/RConn1 -- inv_M2/LConn1
  Three-Phase V-I Measurement1/LConn2 -- inv_M2/RConn2
  Three-Phase V-I Measurement1/LConn3 -- inv_M2/RConn3
  inv_M1/RConn1 -- Three-Phase V-I Measurement/LConn1
  inv_M1/RConn2 -- Three-Phase V-I Measurement/LConn2
  inv_M1/RConn3 -- Three-Phase V-I Measurement/LConn3
  DC Voltage Source/RConn1 -- inv_M1/LConn1
  inv_M1/LConn2 -- DC Voltage Source/LConn1 -- Ground1/LConn1
  Relay_G2/RConn2 -- Relay_G1/RConn2 -- LOAD BANK/LConn2
  Relay_G2/RConn1 -- Relay_G1/RConn1 -- LOAD BANK/LConn1
  Relay_G2/RConn3 -- Relay_G1/RConn3 -- LOAD BANK/LConn3
  Relay_G2/LConn1 -- Three-Phase V-I Measurement2/RConn1
  Relay_G2/LConn2 -- Three-Phase V-I Measurement2/RConn2
  Relay_G2/LConn3 -- Three-Phase V-I Measurement2/RConn3
  Three-Phase V-I Measurement3/RConn1 -- Relay_G1/LConn1
  Three-Phase V-I Measurement3/RConn2 -- Relay_G1/LConn2
  Three-Phase V-I Measurement3/RConn3 -- Relay_G1/LConn3

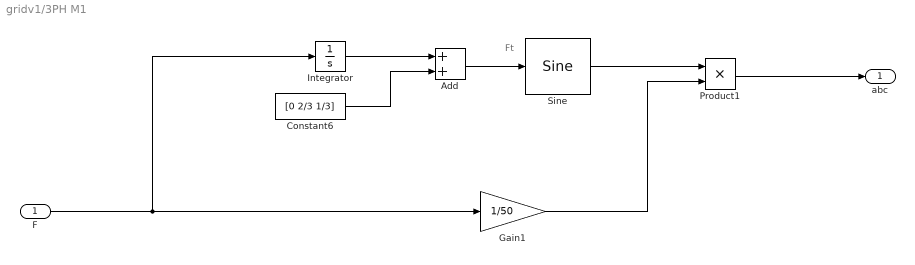
== system gridv1/3PH M1 ==
  note: Ft
  F : Inport
  Add : Sum
  Constant6 : Constant  Value=[0 2/3 1/3]
  Gain1 : Gain  Gain=1/50
  Integrator : Integrator
  Product1 : Product
  Sine : simulink/Lookup Tables/Sine  Formula=sin(2*pi*u)  NumDataPoints=(2^5)+1  OutputWordLength=16  InternalRulePriority=Speed
  abc : Outport
  wires:
  F/1 -> Gain1/1, Integrator/1
  Gain1/1 -> Product1/2
  Sine/1 -> Product1/1
  Product1/1 -> abc/1
  Integrator/1 -> Add/1
  Constant6/1 -> Add/2
  Add/1 -> Sine/1

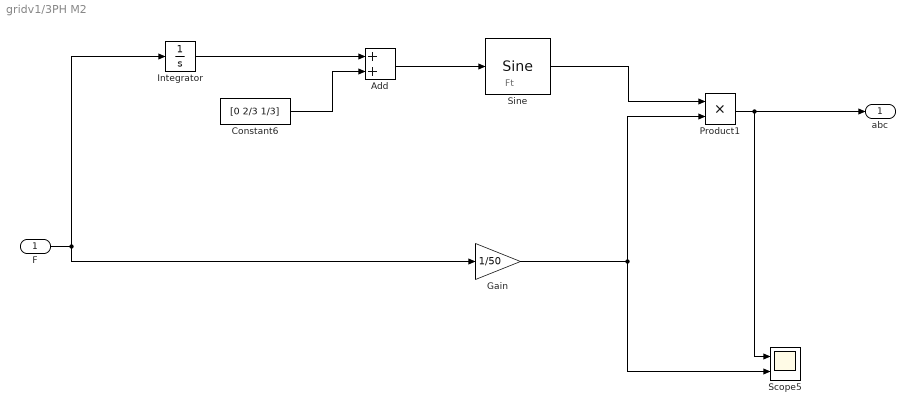
== system gridv1/3PH M2 ==
  note: Ft
  F : Inport
  Add : Sum
  Constant6 : Constant  Value=[0 2/3 1/3]
  Gain : Gain  Gain=1/50
  Integrator : Integrator
  Product1 : Product
  Scope5 : Scope  NumInputPorts=2
  Sine : simulink/Lookup Tables/Sine  Formula=sin(2*pi*u)  NumDataPoints=(2^5)+1  OutputWordLength=16  InternalRulePriority=Speed
  abc : Outport
  wires:
  F/1 -> Gain/1, Integrator/1
  Gain/1 -> Product1/2, Scope5/2
  Sine/1 -> Product1/1
  Product1/1 -> abc/1, Scope5/1
  Integrator/1 -> Add/1
  Constant6/1 -> Add/2
  Add/1 -> Sine/1

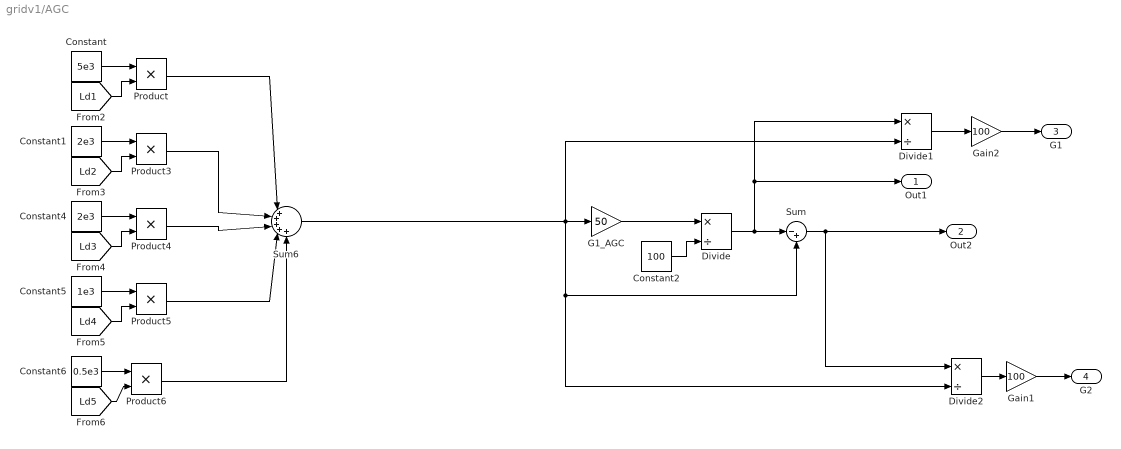
== system gridv1/AGC ==
  Constant : Constant  Value=5e3
  Constant1 : Constant  Value=2e3
  Constant2 : Constant  Value=100
  Constant4 : Constant  Value=2e3
  Constant5 : Constant  Value=1e3
  Constant6 : Constant  Value=0.5e3
  Divide : Product  Inputs=*/
  Divide1 : Product  Inputs=*/
  Divide2 : Product  Inputs=*/
  G1_AGC : Gain  Gain=50
  Gain1 : Gain  Gain=100
  Gain2 : Gain  Gain=100
  Product{,3..6} (5 alike) : Product  OutDataTypeStr=Inherit: Same as first input
  Sum : Sum  Inputs=|-+
  Sum6 : Sum  Inputs=|+++++
  Out1 : Outport
  Out2 : Outport  Port=2
  G1 : Outport  Port=3
  G2 : Outport  Port=4
  wires:
  Constant5/1 -> Product5/1
  [Ld4] -> Product5/2
  Divide/1 -> Divide1/1, Out1/1, Sum/1
  [Ld2] -> Product3/2
  [Ld3] -> Product4/2
  Sum6/1 -> Divide2/2, Sum/2, Divide1/2, G1_AGC/1
  Constant1/1 -> Product3/1
  [Ld1] -> Product/2
  Product5/1 -> Sum6/4
  Constant4/1 -> Product4/1
  Product/1 -> Sum6/1
  [Ld5] -> Product6/2
  Constant6/1 -> Product6/1
  Product3/1 -> Sum6/2
  Constant/1 -> Product/1
  Product6/1 -> Sum6/5
  Product4/1 -> Sum6/3
  Sum/1 -> Divide2/1, Out2/1
  Gain1/1 -> G2/1
  G1_AGC/1 -> Divide/1
  Constant2/1 -> Divide/2
  Divide2/1 -> Gain1/1
  Divide1/1 -> Gain2/1
  Gain2/1 -> G1/1

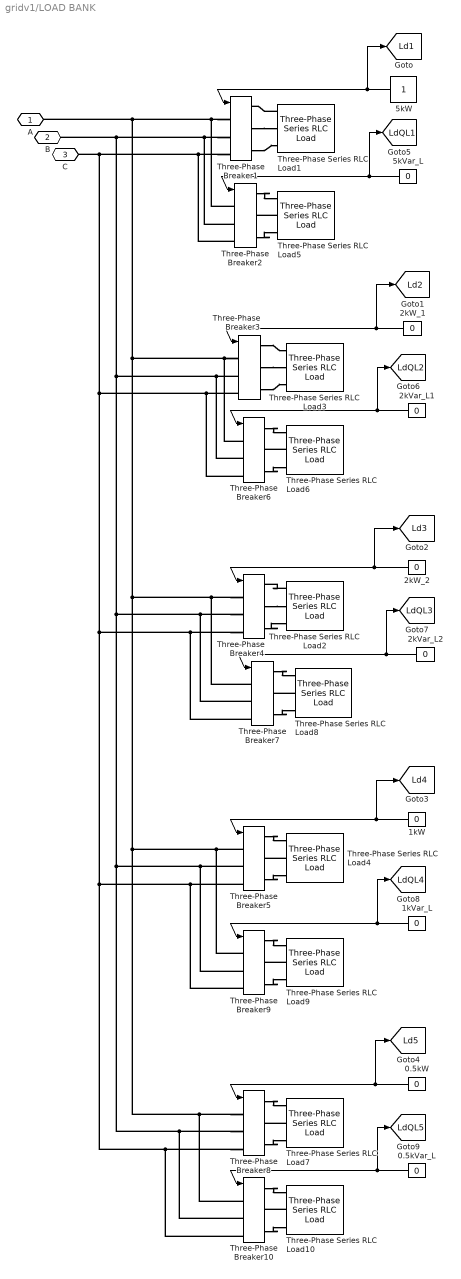
== system gridv1/LOAD BANK ==
  0.5kVar_L : Constant  Value=0
  0.5kW : Constant  Value=0
  1kVar_L : Constant  Value=0
  1kW : Constant  Value=0
  2kVar_L1 : Constant  Value=0
  2kVar_L2 : Constant  Value=0
  2kW_1 : Constant  Value=0
  2kW_2 : Constant  Value=0
  5kVar_L : Constant  Value=0
  5kW : Constant
  Three-Phase Series RLC Load1 : spsThreePhaseSeriesRLCLoadLib/Three-Phase Series RLC Load  LConnTagsString=A|B|C  Configuration=Y (grounded)  NominalVoltage=400  Vabc=[1e3 1e3 1e3]  Vabcp=[1e3 1e3 1e3]  NominalFrequency=50  UnbalancedPower=off  ActivePower=5e3  InductivePower=0  CapacitivePower=0  Pabc=[10e3 9e3 11e3]  QLabc=[100 90 110]  QCabc=[100 90 110]  Pabcp=[10e3 9e3 11e3]  QLabcp=[100 90 110]  QCabcp=[100 90 110]  Measurements=None  LoadType=constant PQ
  Three-Phase Series RLC Load10 : spsThreePhaseSeriesRLCLoadLib/Three-Phase Series RLC Load  LConnTagsString=A|B|C  Configuration=Y (grounded)  NominalVoltage=400  Vabc=[1e3 1e3 1e3]  Vabcp=[1e3 1e3 1e3]  NominalFrequency=50  UnbalancedPower=off  ActivePower=0.5e3/100  InductivePower=0.5e3  CapacitivePower=0  Pabc=[10e3 9e3 11e3]  QLabc=[100 90 110]  QCabc=[100 90 110]  Pabcp=[10e3 9e3 11e3]  QLabcp=[100 90 110]  QCabcp=[100 90 110]  Measurements=None  LoadType=constant PQ
  Three-Phase Series RLC Load2 : spsThreePhaseSeriesRLCLoadLib/Three-Phase Series RLC Load  LConnTagsString=A|B|C  Configuration=Y (grounded)  NominalVoltage=400  Vabc=[1e3 1e3 1e3]  Vabcp=[1e3 1e3 1e3]  NominalFrequency=50  UnbalancedPower=off  ActivePower=2e3  InductivePower=0  CapacitivePower=0  Pabc=[10e3 9e3 11e3]  QLabc=[100 90 110]  QCabc=[100 90 110]  Pabcp=[10e3 9e3 11e3]  QLabcp=[100 90 110]  QCabcp=[100 90 110]  Measurements=None  LoadType=constant PQ
  Three-Phase Series RLC Load3 : spsThreePhaseSeriesRLCLoadLib/Three-Phase Series RLC Load  LConnTagsString=A|B|C  Configuration=Y (grounded)  NominalVoltage=400  Vabc=[1e3 1e3 1e3]  Vabcp=[1e3 1e3 1e3]  NominalFrequency=50  UnbalancedPower=off  ActivePower=2e3  InductivePower=0  CapacitivePower=0  Pabc=[10e3 9e3 11e3]  QLabc=[100 90 110]  QCabc=[100 90 110]  Pabcp=[10e3 9e3 11e3]  QLabcp=[100 90 110]  QCabcp=[100 90 110]  Measurements=None  LoadType=constant PQ
  Three-Phase Series RLC Load4 : spsThreePhaseSeriesRLCLoadLib/Three-Phase Series RLC Load  LConnTagsString=A|B|C  Configuration=Y (grounded)  NominalVoltage=400  Vabc=[1e3 1e3 1e3]  Vabcp=[1e3 1e3 1e3]  NominalFrequency=50  UnbalancedPower=off  ActivePower=1e3  InductivePower=0  CapacitivePower=0  Pabc=[10e3 9e3 11e3]  QLabc=[100 90 110]  QCabc=[100 90 110]  Pabcp=[10e3 9e3 11e3]  QLabcp=[100 90 110]  QCabcp=[100 90 110]  Measurements=None  LoadType=constant Z
  Three-Phase Series RLC Load5 : spsThreePhaseSeriesRLCLoadLib/Three-Phase Series RLC Load  LConnTagsString=A|B|C  Configuration=Y (grounded)  NominalVoltage=400  Vabc=[1e3 1e3 1e3]  Vabcp=[1e3 1e3 1e3]  NominalFrequency=50  UnbalancedPower=off  ActivePower=5e3/100  InductivePower=5e3  CapacitivePower=0  Pabc=[10e3 9e3 11e3]  QLabc=[100 90 110]  QCabc=[100 90 110]  Pabcp=[10e3 9e3 11e3]  QLabcp=[100 90 110]  QCabcp=[100 90 110]  Measurements=None  LoadType=constant PQ
  Three-Phase Series RLC Load6 : spsThreePhaseSeriesRLCLoadLib/Three-Phase Series RLC Load  LConnTagsString=A|B|C  Configuration=Y (grounded)  NominalVoltage=400  Vabc=[1e3 1e3 1e3]  Vabcp=[1e3 1e3 1e3]  NominalFrequency=50  UnbalancedPower=off  ActivePower=2e3/100  InductivePower=2e3  CapacitivePower=0  Pabc=[10e3 9e3 11e3]  QLabc=[100 90 110]  QCabc=[100 90 110]  Pabcp=[10e3 9e3 11e3]  QLabcp=[100 90 110]  QCabcp=[100 90 110]  Measurements=None  LoadType=constant PQ
  Three-Phase Series RLC Load7 : spsThreePhaseSeriesRLCLoadLib/Three-Phase Series RLC Load  LConnTagsString=A|B|C  Configuration=Y (grounded)  NominalVoltage=400  Vabc=[1e3 1e3 1e3]  Vabcp=[1e3 1e3 1e3]  NominalFrequency=50  UnbalancedPower=off  ActivePower=1e3  InductivePower=0  CapacitivePower=0  Pabc=[10e3 9e3 11e3]  QLabc=[100 90 110]  QCabc=[100 90 110]  Pabcp=[10e3 9e3 11e3]  QLabcp=[100 90 110]  QCabcp=[100 90 110]  Measurements=None  LoadType=constant Z
  Three-Phase Series RLC Load8 : spsThreePhaseSeriesRLCLoadLib/Three-Phase Series RLC Load  LConnTagsString=A|B|C  Configuration=Y (grounded)  NominalVoltage=400  Vabc=[1e3 1e3 1e3]  Vabcp=[1e3 1e3 1e3]  NominalFrequency=50  UnbalancedPower=off  ActivePower=2e3/100  InductivePower=2e3  CapacitivePower=0  Pabc=[10e3 9e3 11e3]  QLabc=[100 90 110]  QCabc=[100 90 110]  Pabcp=[10e3 9e3 11e3]  QLabcp=[100 90 110]  QCabcp=[100 90 110]  Measurements=None  LoadType=constant PQ
  Three-Phase Series RLC Load9 : spsThreePhaseSeriesRLCLoadLib/Three-Phase Series RLC Load  LConnTagsString=A|B|C  Configuration=Y (grounded)  NominalVoltage=400  Vabc=[1e3 1e3 1e3]  Vabcp=[1e3 1e3 1e3]  NominalFrequency=50  UnbalancedPower=off  ActivePower=1e3/100  InductivePower=1e3  CapacitivePower=0  Pabc=[10e3 9e3 11e3]  QLabc=[100 90 110]  QCabc=[100 90 110]  Pabcp=[10e3 9e3 11e3]  QLabcp=[100 90 110]  QCabcp=[100 90 110]  Measurements=None  LoadType=constant PQ
  Three-Phase Breaker{1..10} (10 alike) : spsThreePhaseBreakerLib/Three-Phase Breaker  InitialState=closed  SwitchA=on  SwitchB=on  SwitchC=on  SwitchTimes="[1/60  5/60]"  External=on  BreakerResistance=0.01  SnubberResistance=1e6  SnubberCapacitance=inf  Measurements=None
  A : PMIOPort  Side=Left
  B : PMIOPort  Port=2  Side=Left
  C : PMIOPort  Port=3  Side=Left
  tag scope: Ld1=global, Ld2=global, Ld3=global, Ld4=global, Ld5=global, LdQL1=global, LdQL2=global, LdQL3=global, LdQL4=global, LdQL5=global
  wires:
  1kW/1 -> [Ld4], Three-Phase Breaker5/1
  5kW/1 -> [Ld1], Three-Phase Breaker1/1
  2kW_1/1 -> [Ld2], Three-Phase Breaker3/1
  0.5kW/1 -> [Ld5], Three-Phase Breaker8/1
  2kW_2/1 -> [Ld3], Three-Phase Breaker4/1
  5kVar_L/1 -> [LdQL1], Three-Phase Breaker2/1
  2kVar_L1/1 -> [LdQL2], Three-Phase Breaker6/1
  2kVar_L2/1 -> [LdQL3], Three-Phase Breaker7/1
  1kVar_L/1 -> [LdQL4], Three-Phase Breaker9/1
  0.5kVar_L/1 -> [LdQL5], Three-Phase Breaker10/1
  connections:
  Three-Phase Breaker1/LConn2 -- Three-Phase Breaker2/LConn2 -- Three-Phase Breaker6/LConn2 -- Three-Phase Breaker3/LConn2 -- Three-Phase Breaker7/LConn2 -- Three-Phase Breaker4/LConn2 -- Three-Phase Breaker10/LConn2 -- Three-Phase Breaker8/LConn2 -- Three-Phase Breaker9/LConn2 -- Three-Phase Breaker5/LConn2 -- B/RConn1
  Three-Phase Series RLC Load1/LConn1 -- Three-Phase Breaker1/RConn1
  Three-Phase Breaker1/LConn3 -- Three-Phase Breaker2/LConn3 -- Three-Phase Breaker6/LConn3 -- Three-Phase Breaker3/LConn3 -- Three-Phase Breaker7/LConn3 -- Three-Phase Breaker4/LConn3 -- Three-Phase Breaker10/LConn3 -- Three-Phase Breaker8/LConn3 -- Three-Phase Breaker9/LConn3 -- Three-Phase Breaker5/LConn3 -- C/RConn1
  Three-Phase Breaker1/RConn3 -- Three-Phase Series RLC Load1/LConn3
  Three-Phase Series RLC Load2/LConn1 -- Three-Phase Breaker4/RConn1
  Three-Phase Breaker8/LConn1 -- Three-Phase Breaker10/LConn1 -- Three-Phase Breaker9/LConn1 -- Three-Phase Breaker5/LConn1 -- Three-Phase Breaker7/LConn1 -- Three-Phase Breaker4/LConn1 -- Three-Phase Breaker6/LConn1 -- Three-Phase Breaker3/LConn1 -- Three-Phase Breaker2/LConn1 -- Three-Phase Breaker1/LConn1 -- A/RConn1
  Three-Phase Breaker1/RConn2 -- Three-Phase Series RLC Load1/LConn2
  Three-Phase Breaker8/RConn3 -- Three-Phase Series RLC Load7/LConn3
  Three-Phase Breaker4/RConn3 -- Three-Phase Series RLC Load2/LConn3
  Three-Phase Breaker3/RConn2 -- Three-Phase Series RLC Load3/LConn2
  Three-Phase Series RLC Load7/LConn2 -- Three-Phase Breaker8/RConn2
  Three-Phase Breaker8/RConn1 -- Three-Phase Series RLC Load7/LConn1
  Three-Phase Breaker4/RConn2 -- Three-Phase Series RLC Load2/LConn2
  Three-Phase Breaker5/RConn1 -- Three-Phase Series RLC Load4/LConn1
  Three-Phase Breaker5/RConn3 -- Three-Phase Series RLC Load4/LConn3
  Three-Phase Breaker3/RConn3 -- Three-Phase Series RLC Load3/LConn3
  Three-Phase Breaker3/RConn1 -- Three-Phase Series RLC Load3/LConn1
  Three-Phase Series RLC Load4/LConn2 -- Three-Phase Breaker5/RConn2
  Three-Phase Breaker2/RConn3 -- Three-Phase Series RLC Load5/LConn3
  Three-Phase Series RLC Load5/LConn2 -- Three-Phase Breaker2/RConn2
  Three-Phase Breaker2/RConn1 -- Three-Phase Series RLC Load5/LConn1
  Three-Phase Breaker6/RConn1 -- Three-Phase Series RLC Load6/LConn1
  Three-Phase Series RLC Load6/LConn2 -- Three-Phase Breaker6/RConn2
  Three-Phase Breaker6/RConn3 -- Three-Phase Series RLC Load6/LConn3
  Three-Phase Series RLC Load8/LConn2 -- Three-Phase Breaker7/RConn2
  Three-Phase Breaker7/RConn3 -- Three-Phase Series RLC Load8/LConn3
  Three-Phase Breaker7/RConn1 -- Three-Phase Series RLC Load8/LConn1
  Three-Phase Series RLC Load9/LConn2 -- Three-Phase Breaker9/RConn2
  Three-Phase Breaker9/RConn3 -- Three-Phase Series RLC Load9/LConn3
  Three-Phase Breaker9/RConn1 -- Three-Phase Series RLC Load9/LConn1
  Three-Phase Series RLC Load10/LConn2 -- Three-Phase Breaker10/RConn2
  Three-Phase Breaker10/RConn3 -- Three-Phase Series RLC Load10/LConn3
  Three-Phase Breaker10/RConn1 -- Three-Phase Series RLC Load10/LConn1

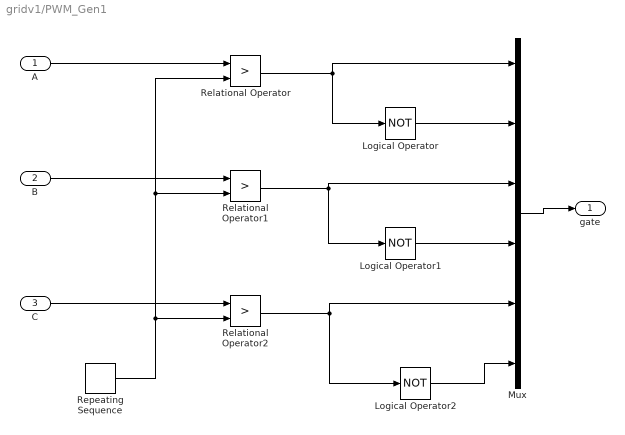
== system gridv1/PWM_Gen1 ==
  A : Inport
  B : Inport  Port=2
  C : Inport  Port=3
  Logical Operator : Logic  Operator=NOT  IconShape=distinctive  AllPortsSameDT=off  OutDataTypeStr=boolean
  Logical Operator1 : Logic  Operator=NOT  IconShape=distinctive  AllPortsSameDT=off  OutDataTypeStr=boolean
  Logical Operator2 : Logic  Operator=NOT  IconShape=distinctive  AllPortsSameDT=off  OutDataTypeStr=boolean
  Mux : Mux  Inputs=6
  Relational Operator : RelationalOperator  Operator=>  OutDataTypeStr=boolean  RndMeth=Nearest
  Relational Operator1 : RelationalOperator  Operator=>  OutDataTypeStr=boolean  RndMeth=Nearest
  Relational Operator2 : RelationalOperator  Operator=>  OutDataTypeStr=boolean  RndMeth=Nearest
  Repeating Sequence : simulink/Sources/Repeating Sequence  rep_seq_t=[0 0.5/5000 1/5000]  rep_seq_y=[-1 1 -1]
  gate : Outport
  wires:
  A/1 -> Relational Operator/1
  C/1 -> Relational Operator2/1
  Repeating Sequence/1 -> Relational Operator1/2, Relational Operator/2, Relational Operator2/2
  B/1 -> Relational Operator1/1
  Relational Operator/1 -> Logical Operator/1, Mux/1
  Logical Operator/1 -> Mux/2
  Relational Operator1/1 -> Logical Operator1/1, Mux/3
  Logical Operator1/1 -> Mux/4
  Relational Operator2/1 -> Logical Operator2/1, Mux/5
  Logical Operator2/1 -> Mux/6
  Mux/1 -> gate/1

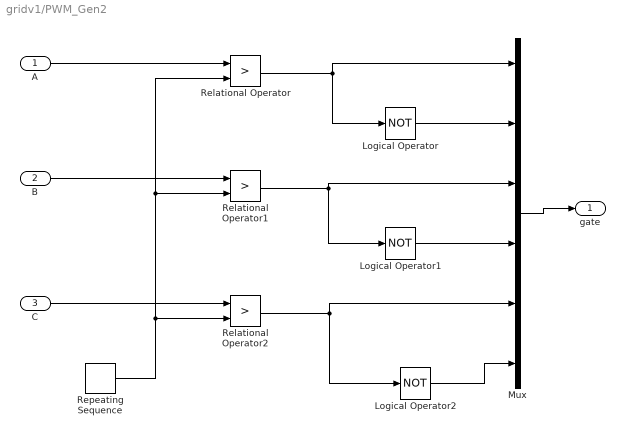
== system gridv1/PWM_Gen2 ==
  A : Inport
  B : Inport  Port=2
  C : Inport  Port=3
  Logical Operator : Logic  Operator=NOT  IconShape=distinctive  AllPortsSameDT=off  OutDataTypeStr=boolean
  Logical Operator1 : Logic  Operator=NOT  IconShape=distinctive  AllPortsSameDT=off  OutDataTypeStr=boolean
  Logical Operator2 : Logic  Operator=NOT  IconShape=distinctive  AllPortsSameDT=off  OutDataTypeStr=boolean
  Mux : Mux  Inputs=6
  Relational Operator : RelationalOperator  Operator=>  OutDataTypeStr=boolean  RndMeth=Nearest
  Relational Operator1 : RelationalOperator  Operator=>  OutDataTypeStr=boolean  RndMeth=Nearest
  Relational Operator2 : RelationalOperator  Operator=>  OutDataTypeStr=boolean  RndMeth=Nearest
  Repeating Sequence : simulink/Sources/Repeating Sequence  rep_seq_t=[0 0.5/5000 1/5000]  rep_seq_y=[-1 1 -1]
  gate : Outport
  wires:
  A/1 -> Relational Operator/1
  C/1 -> Relational Operator2/1
  Repeating Sequence/1 -> Relational Operator1/2, Relational Operator/2, Relational Operator2/2
  B/1 -> Relational Operator1/1
  Relational Operator/1 -> Logical Operator/1, Mux/1
  Logical Operator/1 -> Mux/2
  Relational Operator1/1 -> Logical Operator1/1, Mux/3
  Logical Operator1/1 -> Mux/4
  Relational Operator2/1 -> Logical Operator2/1, Mux/5
  Logical Operator2/1 -> Mux/6
  Mux/1 -> gate/1

== system gridv1/Parrallel Op ON ==
  Data Store Read : DataStoreRead  DataStoreName=synch1_  IndexOptions=Index vector (dialog)  Indices=1  OutputSizes=1
  Data Store Read1 : DataStoreRead  DataStoreName=synch2_  IndexOptions=Index vector (dialog)  Indices=1  OutputSizes=1
  Logical Operator : Logic  AllPortsSameDT=off  OutDataTypeStr=boolean
  Out1 : Outport
  wires:
  Data Store Read1/1 -> Logical Operator/2
  Logical Operator/1 -> Out1/1
  Data Store Read/1 -> Logical Operator/1

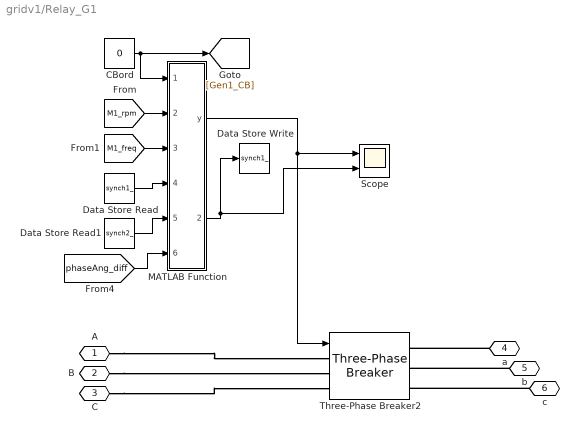
== system gridv1/Relay_G1 ==
  CBord : Constant  Value=0
  Data Store Read : DataStoreRead  DataStoreName=synch1_  IndexOptions=Index vector (dialog)  Indices=1  OutputSizes=1
  Data Store Read1 : DataStoreRead  DataStoreName=synch2_  IndexOptions=Index vector (dialog)  Indices=1  OutputSizes=1
  Data Store Write : DataStoreWrite  DataStoreName=synch1_  IndexOptions=Index vector (dialog)  Indices=1  OutputSizes=1
  MATLAB Function : MATLAB Function  TreatAsAtomicUnit=on
  Scope : Scope  NumInputPorts=2
  Three-Phase Breaker2 : spsThreePhaseBreakerLib/Three-Phase Breaker  InitialState=closed  SwitchA=on  SwitchB=on  SwitchC=on  SwitchTimes="[1/60  5/60]"  External=on  BreakerResistance=0.01  SnubberResistance=1e6  SnubberCapacitance=inf  Measurements=None
  A : PMIOPort  Side=Left
  B : PMIOPort  Port=2  Side=Left
  C : PMIOPort  Port=3  Side=Left
  a : PMIOPort  Port=4  Side=Right
  b : PMIOPort  Port=5  Side=Right
  c : PMIOPort  Port=6  Side=Right
  wires:
  MATLAB Function/1(y) -> Three-Phase Breaker2/1, Scope/1
  [M1_rpm] -> MATLAB Function/2(rpm)
  CBord/1 -> [Gen1_CB], MATLAB Function/1(CBord)
  Data Store Read/1 -> MATLAB Function/4(sync1)
  MATLAB Function/2(sync) -> Data Store Write/1, Scope/2
  [M1_freq] -> MATLAB Function/3(freq1)
  [phaseAng_diff] -> MATLAB Function/6(delta_phase)
  Data Store Read1/1 -> MATLAB Function/5(sync2)
  connections:
  c/RConn1 -- Three-Phase Breaker2/RConn3
  a/RConn1 -- Three-Phase Breaker2/RConn1
  b/RConn1 -- Three-Phase Breaker2/RConn2
  A/RConn1 -- Three-Phase Breaker2/LConn1
  B/RConn1 -- Three-Phase Breaker2/LConn2
  C/RConn1 -- Three-Phase Breaker2/LConn3

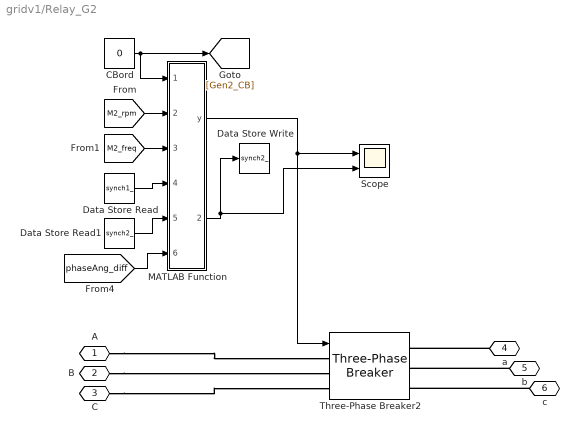
== system gridv1/Relay_G2 ==
  CBord : Constant  Value=0
  Data Store Read : DataStoreRead  DataStoreName=synch1_  IndexOptions=Index vector (dialog)  Indices=1  OutputSizes=1
  Data Store Read1 : DataStoreRead  DataStoreName=synch2_  IndexOptions=Index vector (dialog)  Indices=1  OutputSizes=1
  Data Store Write : DataStoreWrite  DataStoreName=synch2_  IndexOptions=Index vector (dialog)  Indices=1  OutputSizes=1
  MATLAB Function : MATLAB Function  TreatAsAtomicUnit=on
  Scope : Scope  NumInputPorts=2
  Three-Phase Breaker2 : spsThreePhaseBreakerLib/Three-Phase Breaker  InitialState=closed  SwitchA=on  SwitchB=on  SwitchC=on  SwitchTimes="[1/60  5/60]"  External=on  BreakerResistance=0.01  SnubberResistance=1e6  SnubberCapacitance=inf  Measurements=None
  A : PMIOPort  Side=Left
  B : PMIOPort  Port=2  Side=Left
  C : PMIOPort  Port=3  Side=Left
  a : PMIOPort  Port=4  Side=Right
  b : PMIOPort  Port=5  Side=Right
  c : PMIOPort  Port=6  Side=Right
  wires:
  MATLAB Function/1(y) -> Three-Phase Breaker2/1, Scope/1
  [M2_rpm] -> MATLAB Function/2(rpm)
  CBord/1 -> [Gen2_CB], MATLAB Function/1(CBord)
  Data Store Read/1 -> MATLAB Function/4(sync1)
  MATLAB Function/2(sync) -> Data Store Write/1, Scope/2
  [M2_freq] -> MATLAB Function/3(freq1)
  [phaseAng_diff] -> MATLAB Function/6(delta_phase)
  Data Store Read1/1 -> MATLAB Function/5(sync2)
  connections:
  c/RConn1 -- Three-Phase Breaker2/RConn3
  a/RConn1 -- Three-Phase Breaker2/RConn1
  b/RConn1 -- Three-Phase Breaker2/RConn2
  A/RConn1 -- Three-Phase Breaker2/LConn1
  B/RConn1 -- Three-Phase Breaker2/LConn2
  C/RConn1 -- Three-Phase Breaker2/LConn3

== system gridv1/Subsystem ==
  In1 : Inport
  Constant1 : Constant  Value=10e3
  Constant3 : Constant  Value=1500
  Divide : Product  Inputs=*/
  Gain12 : Gain  Gain=9.5488
  MATLAB Function : MATLAB Function  TreatAsAtomicUnit=on
  Out1 : Outport
  wires:
  Gain12/1 -> Divide/1
  Divide/1 -> Out1/1
  Constant3/1 -> Divide/2
  MATLAB Function/1(y) -> Gain12/1
  In1/1 -> MATLAB Function/1(u)
  Constant1/1 -> MATLAB Function/2(mech)
